simulink model "Speedgoat_V32"  (R2024b)
settings: Solver=FixedStepDiscrete  StartTime=0.0  StopTime=inf  FixedStep=0.001  RelTol=1e-3  EnableMultiTasking=on
model workspace (MAT data in the model file):
  Test = 10000000
undefined symbols (not defined in the file): CAN, Down, dspblkCoreblockFVToolHelper, FD, gcbh, IO397, Pull
libraries: speedgoatlib_fpga x6, speedgoatlib_fpga_dio x3, speedgoatlib_IO691 x1, speedgoatlib_fpga_analog_io x1, simulink x1
(part 2 of 2)

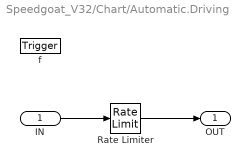
== system Speedgoat_V32/Chart/Automatic.Driving ==
  IN : Inport  OutMin=[1]  OutMax=[4]  OutDataTypeStr=double  PortDimensions=1
  f : TriggerPort  TriggerType=function-call  VariantControl=(inherit)  SampleTimeType=periodic  SampleTime=0.001
      settings: CopyFcn=Stateflow.SLINSF.SimulinkMan.removeBlockPreDeleteFcn  PreDeleteFcn=Stateflow.SLINSF.SimulinkMan.unsafePredeleteFcn
  Rate Limiter : RateLimiter  RisingSlewLimit=0.5  FallingSlewLimit=-0.5  SampleTimeMode=inherited  InitialCondition=1
  OUT : Outport  OutMin=[1]  OutMax=[4]  OutputWhenDisabled=reset  InitialOutput=[1]
  wires:
  Rate Limiter/1 -> OUT/1
  IN/1 -> Rate Limiter/1

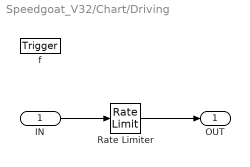
== system Speedgoat_V32/Chart/Driving ==
  IN : Inport  OutMin=[1]  OutMax=[4]  OutDataTypeStr=double  PortDimensions=1
  f : TriggerPort  TriggerType=function-call  VariantControl=(inherit)  SampleTimeType=periodic  SampleTime=0.001
      settings: CopyFcn=Stateflow.SLINSF.SimulinkMan.removeBlockPreDeleteFcn  PreDeleteFcn=Stateflow.SLINSF.SimulinkMan.unsafePredeleteFcn
  Rate Limiter : RateLimiter  RisingSlewLimit=0.5  FallingSlewLimit=-0.5  SampleTimeMode=inherited  InitialCondition=1
  OUT : Outport  OutMin=[1]  OutMax=[4]  OutputWhenDisabled=reset  InitialOutput=[1]
  wires:
  Rate Limiter/1 -> OUT/1
  IN/1 -> Rate Limiter/1

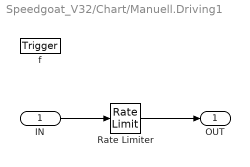
== system Speedgoat_V32/Chart/Manuell.Driving1 ==
  IN : Inport  OutMin=[1]  OutMax=[4]  OutDataTypeStr=double  PortDimensions=1
  f : TriggerPort  TriggerType=function-call  VariantControl=(inherit)  SampleTimeType=periodic  SampleTime=0.001
      settings: CopyFcn=Stateflow.SLINSF.SimulinkMan.removeBlockPreDeleteFcn  PreDeleteFcn=Stateflow.SLINSF.SimulinkMan.unsafePredeleteFcn
  Rate Limiter : RateLimiter  RisingSlewLimit=0.5  FallingSlewLimit=-0.5  SampleTimeMode=inherited  InitialCondition=1
  OUT : Outport  OutMin=[1]  OutMax=[4]  OutputWhenDisabled=reset  InitialOutput=[1]
  wires:
  Rate Limiter/1 -> OUT/1
  IN/1 -> Rate Limiter/1

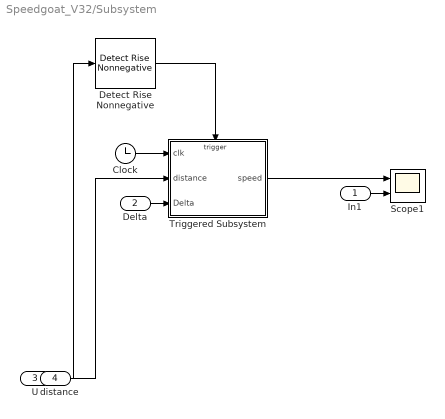
== system Speedgoat_V32/Subsystem ==
  In1 : Inport
  Delta : Inport  Port=2
  U : Inport  Port=3
  distance : Inport  Port=4
  Clock : Clock
  Detect Rise Nonnegative : simulink/Logic and Bit Operations/Detect Rise Nonnegative  vinit=0  OutDataTypeStr=boolean
  Scope1 : Scope  NumInputPorts=2
  Triggered Subsystem : Subsystem  TreatAsAtomicUnit=on
  wires:
  Triggered Subsystem/1(speed) -> Scope1/1
  Detect Rise Nonnegative/1 -> Triggered Subsystem/Trigger
  Delta/1 -> Triggered Subsystem/3(Delta)
  Clock/1 -> Triggered Subsystem/1(clk)
  In1/1 -> Scope1/2
  distance/1 -> Triggered Subsystem/2(distance)
  U/1 -> Detect Rise Nonnegative/1

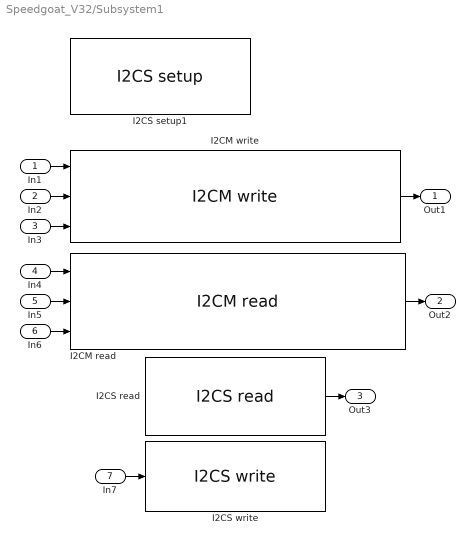
== system Speedgoat_V32/Subsystem1 ==
  In1 : Inport
  In2 : Inport  Port=2
  In3 : Inport  Port=3
  In4 : Inport  Port=4
  In5 : Inport  Port=5
  In6 : Inport  Port=6
  In7 : Inport  Port=7
  I2CM read : speedgoatlib_fpga/I2C/I2CM read  id=1  chan=1  ts=0.001  clockDivider=350  readPrevValue=off  subIndexConfiguration=on  showAckErrorPort=off
      settings: SourceProductName=IO3xx
  I2CM write : speedgoatlib_fpga/I2C/I2CM write  id=1  chan=1  ts=0.001  clockDivider=350  showAckErrorPort=on  readPrevValue=off
      settings: SourceProductName=IO3xx
  I2CS read : speedgoatlib_fpga/I2C/I2CS read  id=1  chan=[1]  regs=[1]  ts=0.001  showDataValidPort=off  showLastRegPort=off  showLastRegValidPort=off
      settings: SourceProductName=IO3xx
  I2CS setup1 : speedgoatlib_fpga/I2C/I2CS setup  id=1  chan=1  slaveID=1  skipRegAddress=off  ts=-1
      settings: SourceProductName=IO3xx
  I2CS write : speedgoatlib_fpga/I2C/I2CS write  id=1  chan=[1]  regs=[1]  ts=0.001
      settings: SourceProductName=IO3xx
  Out1 : Outport
  Out2 : Outport  Port=2
  Out3 : Outport  Port=3
  wires:
  In4/1 -> I2CM read/1
  In1/1 -> I2CM write/1
  In5/1 -> I2CM read/2
  In6/1 -> I2CM read/3
  I2CM read/1 -> Out2/1
  In3/1 -> I2CM write/3
  In2/1 -> I2CM write/2
  I2CS read/1 -> Out3/1
  In7/1 -> I2CS write/1
  I2CM write/1 -> Out1/1

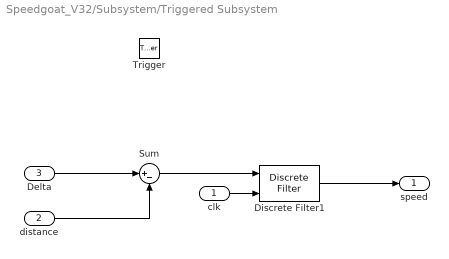
== system Speedgoat_V32/Subsystem/Triggered Subsystem ==
  clk : Inport
  distance : Inport  Port=2
  Delta : Inport  Port=3
  Trigger : TriggerPort  VariantControl=(inherit)
  Discrete Filter1 : DiscreteFilter  LoadFcn=dspblkCoreblockFVToolHelper(gcbh,'load');  ExternalReset=Rising
      settings: CopyFcn=dspblkCoreblockFVToolHelper(gcbh,'copy');  DeleteFcn=dspblkCoreblockFVToolHelper(gcbh,'close');  ModelCloseFcn=dspblkCoreblockFVToolHelper(gcbh,'close');  PreSaveFcn=dspblkCoreblockFVToolHelper(gcbh,'presave');  PostSaveFcn=dspblkCoreblockFVToolHelper(gcbh,'postsave');  CloseFcn=dspblkCoreblockFVToolHelper(gcbh,'close');  InputPortMap=u0,r7
  Sum : Sum  Inputs=|+-
  speed : Outport
  wires:
  Delta/1 -> Sum/1
  distance/1 -> Sum/2
  Sum/1 -> Discrete Filter1/1
  Discrete Filter1/1 -> speed/1
  clk/1 -> Discrete Filter1/2

== stateflow chart Speedgoat_V32/Chart ==
  state Manuell
    state OUT = Driving1(IN) [function]
    state Emergency_stop
      du: speed_out = Driving1(RESET);
      du: break_motor_out = 5;
      du: break_mechanically_out = 5;
      du: direction_out = 5;
      du: cruise_out = 5;
      du: emergency_stop_out = 5;
    state Vorwaerts [group]
      state V_schnell
        du: speed_out = Driving1(3);
        du: break_motor_out = 1;
        du: break_mechanically_out = 0;
        du: direction_out = 5;
        du: cruise_out = 5;
        du: emergency_stop_out = 0;
      state V_langsam
        du: speed_out = Driving1(1.5);
        du: break_motor_out = 1;
        du: break_mechanically_out = 0;
        du: direction_out = 5;
        du: cruise_out = 5;
        du: emergency_stop_out = 0;
      V_schnell -> V_langsam [order 2] : [manual_mod == 5]
      V_langsam -> V_schnell [order 2] : [manual_mod == 4]
    state Manual
      du: speed_out = 1;
      du: Driving1(RESET);
      du: break_motor_out = 5;
      du: direction_out = 5;
      du: cruise_out = 5;
      du: break_mechanically_out = 0;
      du: emergency_stop_out = 0;
    state Collector_manual_in_0_
    state Rueckwaerts [group]
      state R_langsam
        du: speed_out = Driving1(1.5);
        du: break_motor_out = 1;
        du: break_mechanically_out = 0;
        du: direction_out = 0;
        du: cruise_out = 5;
        du: emergency_stop_out = 0;
      state R_schnell
        du: speed_out = Driving1(3);
        du: break_motor_out = 1;
        du: break_mechanically_out = 0;
        du: direction_out = 0;
        du: cruise_out = 5;
        du: emergency_stop_out = 0;
      R_schnell -> R_langsam [order 2] : [manual_mod == 2]
      R_langsam -> R_schnell [order 2] : [manual_mod == 1]
    state Emergency_stop1
      du: speed_out = Driving1(RESET);
      du: break_motor_out = 5;
      du: break_mechanically_out = 5;
      du: direction_out = 5;
      du: cruise_out = 5;
      du: emergency_stop_out = 5;
    V_schnell -> Manuell.Emergency_stop [order 1] : [emergency_stop_in == 1]
    V_langsam -> Manuell.Emergency_stop [order 1] : [emergency_stop_in == 1]
    Manual -> Manuell.Emergency_stop [order 1] : [emergency_stop_in == 1]
    Manuell.Emergency_stop -> Manual : [reset_in == 1]
    Manual -> V_langsam [order 2] : [manual_mod == 4]
    V_schnell -> Collector_manual_in_0_ [order 3] : [manual_in == 0]
    V_langsam -> Collector_manual_in_0_ [order 4] : [manual_in == 0]
    V_schnell -> Manual [order 4] : [manual_mod == 3]
    V_langsam -> Manual [order 3] : [manual_mod == 3]
    R_langsam -> Collector_manual_in_0_ [order 4] : [manual_in == 0]
    R_schnell -> Manual [order 4] : [manual_mod == 3]
    R_langsam -> Manual [order 3] : [manual_mod == 3]
    R_schnell -> Collector_manual_in_0_ [order 3] : [manual_in == 0]
    Manual -> R_langsam [order 3] : [manual_mod == 2]
    Manual -> Emergency_stop1 [order 5] : [emergency_stop_in == 1]
    Emergency_stop1 -> Manual : [reset_in == 1]
    R_langsam -> Emergency_stop1 [order 1] : [emergency_stop_in == 1]
    R_schnell -> Emergency_stop1 [order 1] : [emergency_stop_in == 1]
  state OUT = Driving(IN) [function]
  state Automatic [group]
    state OUT = Driving(IN) [function]
    state Stop
      du: speed_out = Driving(RESET);
      du: break_motor_out = 1;
      du: break_mechanically_out = 0;
      du: direction_out = 5;
      du: cruise_out = 5;
      du: emergency_stop_out = 0;
    state Emergency_stop
      du: speed_out = Driving(RESET);
      du: break_motor_out = 5;
      du: break_mechanically_out = 5;
      du: direction_out = 5;
      du: cruise_out = 5;
      du: emergency_stop_out = 5;
    state Automatic
      du: speed_out = 1;
      du: Driving(RESET);
      du: break_motor_out = 5;
      du: direction_out = 5;
      du: cruise_out = 5;
      du: break_mechanically_out = 0;
      du: emergency_stop_out = 0;
    state Drive
      du: speed_out = Driving(speed_in);
      du: break_motor_out = 1;
      du: break_mechanically_out = 0;
      du: direction_out = 5;
      du: cruise_out = 5;
      du: emergency_stop_out = 0;
    state Distance
      du: speed_out = ((distance_in)*(speed_in-1)/distance)+1;
      du: Driving(distance_in);
      du: break_motor_out = 1;
      du: break_mechanically_out = 0;
      du: direction_out = 5;
      du: cruise_out = 5;
      du: emergency_stop_out = 0;
    Distance -> Stop [order 3] : [stop_in == 1]
    Stop -> Automatic.Automatic : [speed_out == 1]
    Drive -> Stop [order 2] : [stop_in == 1]
    Distance -> Automatic.Emergency_stop [order 1] : [emergency_stop_in == 1]
    Automatic.Emergency_stop -> Automatic.Automatic : [reset_in == 1]
    Automatic.Automatic -> Automatic.Emergency_stop [order 1] : [emergency_stop_in == 1]
    Drive -> Automatic.Emergency_stop [order 1] : [emergency_stop_in == 1]
    Automatic.Automatic -> Drive [order 2] : [start_in == 1]
    Drive -> Distance [order 3] : [distance_in < distance]
    Distance -> Drive [order 4] : [distance_in > distance]
    Distance -> Automatic.Automatic [order 2] : [speed_out == 1]
  state Emergency_stop
    du: speed_out = Driving(RESET);
    du: break_motor_out = 5;
    du: break_mechanically_out = 5;
    du: direction_out = 5;
    du: cruise_out = 5;
    du: emergency_stop_out = 5;
  state IDLE
    du: speed_out = 1;
    du: Driving(RESET);
    du: break_motor_out = 5;
    du: direction_out = 5;
    du: cruise_out = 5;
    du: break_mechanically_out = 5;
    du: emergency_stop_out = 0;
  Emergency_stop -> IDLE : [reset_in == 1]
  IDLE -> Emergency_stop [order 1] : [emergency_stop_in == 1]
  (default) -> IDLE
  IDLE -> Manual [order 2] : [manual_in == 1 ]
  Automatic.Automatic -> IDLE [order 3] : [manual_in == 1 ]
  Manual -> IDLE [order 4] : [manual_in == 0]
  IDLE -> Automatic.Automatic [order 3] : [manual_in == 0]
  Collector_manual_in_0_ -> IDLE : [manual_in == 0]
  Drive -> IDLE [order 4] : [manual_in == 1 ]
  data: IN function_input double size=1; OUT function_output; IN function_input double size=1; OUT function_output; IN function_input double size=1; OUT function_output; speed_out output; speed_in input; distance_in input; start_in input; stop_in input; reset_in input; manual_in input; manual_mod input; break_motor_out output; emergency_stop_in input; direction_out output; cruise_out output; break_mechanically_out output; emergency_stop_out output; RESET constant double =1; distance constant double =10
